simulink model "LeadController_Quantized"  (R2021b)
settings: Solver=VariableStepAuto  StartTime=0.0  StopTime=30  RelTol=1e-3
model workspace (MAT data in the model file):
  L = 0.2
values from neighbouring files (symbols this model uses):
  g = 9.81    [simConstants.m]
  Td = 50e-6    (= 5e-05)    [simConstants.m]
  theta0 = deg2rad(5)    [simConstants.m]
libraries: simulink_extras x1
settings Model: Creator=logan  LastModifiedBy=logan

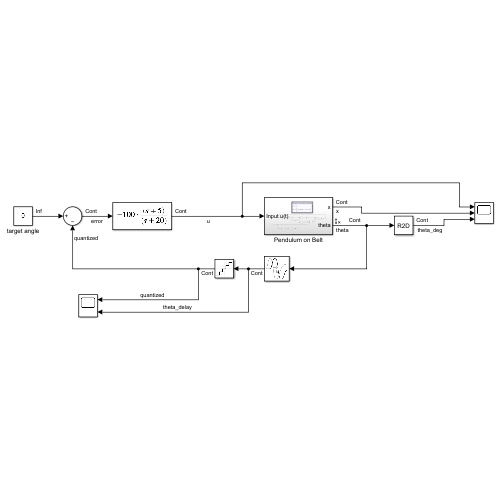
[thumbnail: Simulink's stored preview of the top-level diagram]
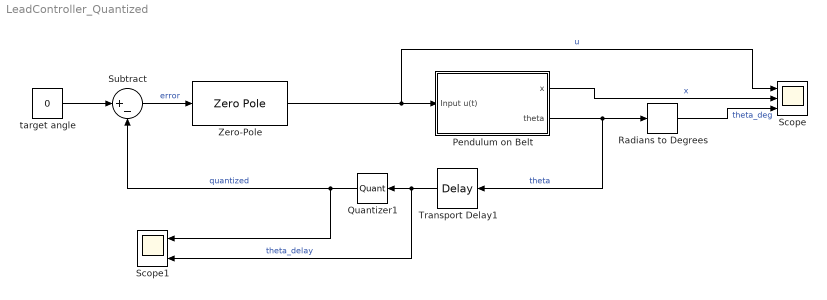
== system LeadController_Quantized ==
  Pendulum on Belt : Subsystem
  Quantizer1 : Quantizer  QuantizationInterval=2*pi/2400
  Radians to Degrees : simulink_extras/Transformations/Radians to Degrees
  Scope : Scope  NumInputPorts=3
  Scope1 : Scope  NumInputPorts=2
  Subtract : Sum  Inputs=|+-
  Transport Delay1 : TransportDelay  DelayTime=Td  InitialOutput=theta0
  Zero-Pole : ZeroPole  Zeros=-5  Poles=-20  Gain=-100
  target angle : Constant  Value=0  OutDataTypeStr=Inherit: Inherit via back propagation
  wires:
  Pendulum on Belt/1(x) -> Scope/2  "x"
  Pendulum on Belt/2(theta) -> Radians to Degrees/1, Transport Delay1/1  "theta"
  Radians to Degrees/1 -> Scope/3  "theta_deg"
  Transport Delay1/1 -> Scope1/2, Quantizer1/1  "theta_delay"
  Subtract/1 -> Zero-Pole/1  "error"
  target angle/1 -> Subtract/1
  Zero-Pole/1 -> Pendulum on Belt/1(Input u(t)), Scope/1  "u"
  Quantizer1/1 -> Subtract/2, Scope1/1  "quantized"

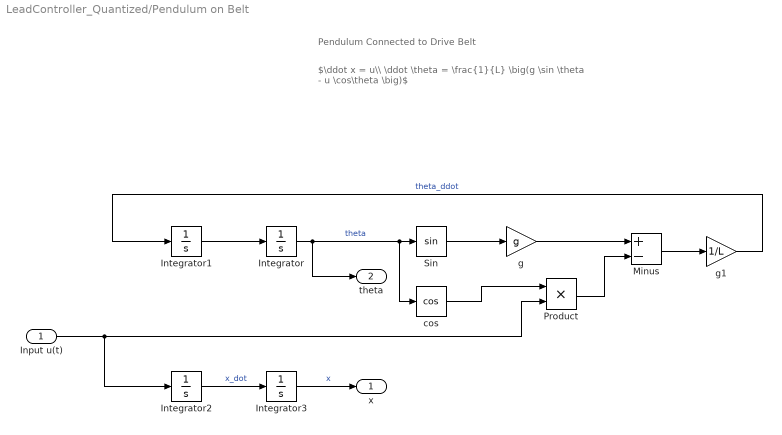
== system LeadController_Quantized/Pendulum on Belt ==
  note: Pendulum Connected to Drive Belt
  note: $\ddot x = u\\ \ddot \theta = \frac{1}{L} \big(g \sin \theta - u \cos\theta \big)$
  Input u(t) : Inport
  Integrator : Integrator  InitialCondition=theta0
  Integrator1 : Integrator
  Integrator2 : Integrator
  Integrator3 : Integrator
  Minus : Sum  Inputs=+-
  Product : Product
  Sin : Trigonometry
  cos : Trigonometry  Operator=cos
  g : Gain  Gain=g
  g1 : Gain  Gain=1/L
  x : Outport
  theta : Outport  Port=2
  wires:
  Integrator/1 -> theta/1, cos/1, Sin/1  "theta"
  Integrator1/1 -> Integrator/1
  Input u(t)/1 -> Integrator2/1, Product/2
  g/1 -> Minus/1
  Sin/1 -> g/1
  cos/1 -> Product/1
  Integrator3/1 -> x/1  "x"
  Product/1 -> Minus/2
  Minus/1 -> g1/1
  g1/1 -> Integrator1/1  "theta_ddot"
  Integrator2/1 -> Integrator3/1  "x_dot"
